simulink model "RC_H10"  (R2025a)
settings: Solver=VariableStepAuto  StartTime=0.0  StopTime=2e-3  MaxStep=5.3e-6/25  RelTol=1e-3
libraries: MK_H x3
settings Model: Creator=Szalay  LastModifiedBy=Szalay

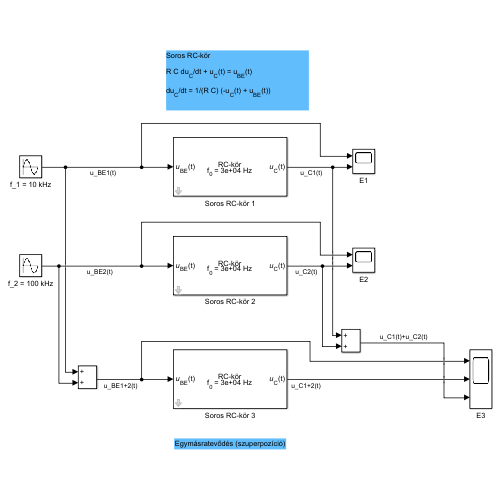
[thumbnail: Simulink's stored preview of the top-level diagram]
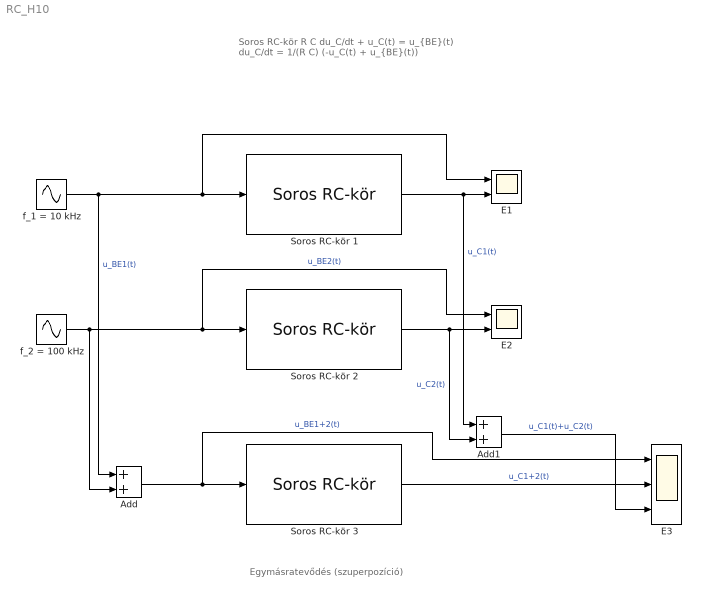
== system RC_H10 ==
  note: Egymásratevődés (szuperpozíció)
  note: Soros RC-kör
      |
      | R C du_C/dt + u_C(t) = u_{BE}(t)
      |
      | du_C/dt = 1/(R C) (-u_C(t) + u_{BE}(t))
  Add : Sum
  Add1 : Sum
  E1 : Scope  NumInputPorts=2
      settings: ActiveDisplayYMinimum=-1.2499998578777105  ActiveDisplayYMaximum=1.2499999842086345
  E2 : Scope  NumInputPorts=2
      settings: ActiveDisplayYMinimum=-1.25  ActiveDisplayYMaximum=1.25
  E3 : Scope  NumInputPorts=3
      settings: ActiveDisplayYMinimum=-2.4847588320173273  ActiveDisplayYMaximum=2.4847567438313813  DataLoggingVariableName=ScopeData2
  Soros RC-kör 1 : MK_H/Soros RC-kör  R=1  C=5.3e-6  u_C0=0
  Soros RC-kör 2 : MK_H/Soros RC-kör  R=1  C=5.3e-6  u_C0=0
  Soros RC-kör 3 : MK_H/Soros RC-kör  R=1  C=5.3e-6  u_C0=0
  f_1 = 10 kHz : Sin  Frequency=2*pi*10000  SampleTime=0
  f_2 = 100 kHz : Sin  Frequency=2*pi*100000  SampleTime=0
  wires:
  f_1 = 10 kHz/1 -> E1/1, Soros RC-kör 1/1, Add/1  "u_BE1(t)"
  Soros RC-kör 1/1 -> Add1/1, E1/2  "u_C1(t)"
  Soros RC-kör 2/1 -> Add1/2, E2/2  "u_C2(t)"
  f_2 = 100 kHz/1 -> Soros RC-kör 2/1, E2/1, Add/2  "u_BE2(t)"
  Add/1 -> E3/1, Soros RC-kör 3/1  "u_BE1+2(t)"
  Soros RC-kör 3/1 -> E3/2  "u_C1+2(t)"
  Add1/1 -> E3/3  "u_C1(t)+u_C2(t)"
